simulink model "phdMain"  (R2023b)
settings: Solver=ode4  StartTime=0.0  StopTime=t.Data(end)  FixedStep=1e-3  RelTol=1e-3
values from neighbouring files (symbols this model uses):
  Am = T * Ac * inv(T)    [ref_model_mrac.m]
  Bm = T * Bc    [ref_model_mrac.m]
  Cm = eye(3)    [ref_model_mrac.m]
  Dm = zeros(3,1)    [ref_model_mrac.m]
undefined symbols (not defined in the file or in its folder): A_bar, AEFF, B_E, C_bar, C_T, Cd_neg, Cd_pos, DiscIntNeverNeededParam, Gamma, H, k, K, L_gain, L_STROKE, M, m3PsToLpm, P_return_Pa, P_supply_Pa, PA_Pa, PaToBar, PB_Pa, RHO, Ts, V01, V02, V_DEAD, v_mPs, W, xc_dot, xc_m
(part 2 of 3)

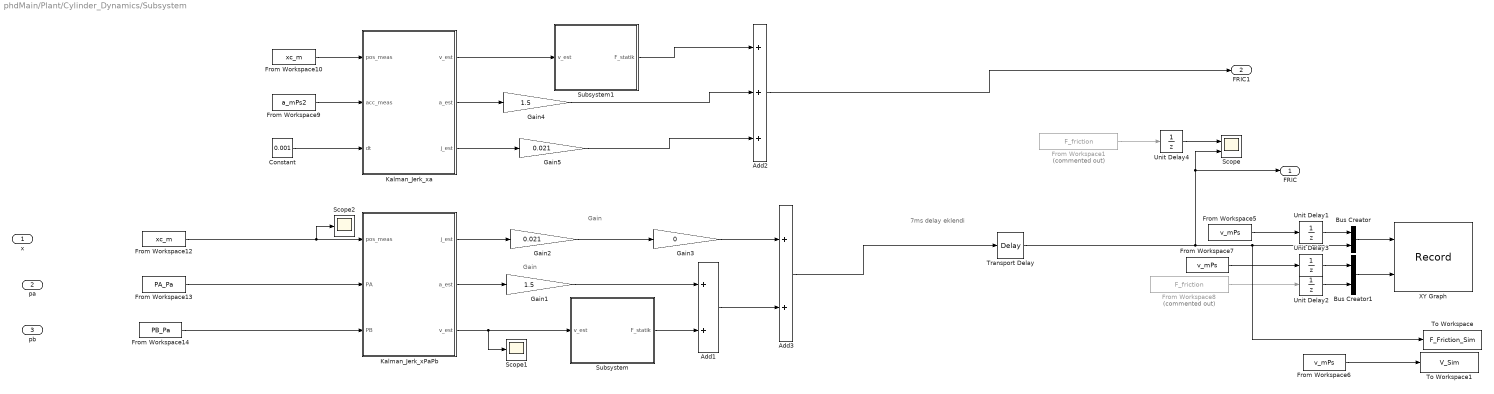
== system phdMain/Plant/Cylinder_Dynamics/Subsystem ==
  note: Gain
  note: 7ms delay eklendi
  note: Gain
  x : Inport
  pa : Inport  Port=2
  pb : Inport  Port=3
  Add1 : Sum
  Add2 : Sum  Inputs=+++
  Add3 : Sum
  Bus Creator : BusCreator  Inputs=2
  Bus Creator1 : BusCreator  Inputs=2
  Constant : Constant  Value=0.001
  From Workspace1 : FromWorkspace  Commented=on  VariableName=F_friction
  From Workspace10 : FromWorkspace  VariableName=xc_m
  From Workspace12 : FromWorkspace  VariableName=xc_m
  From Workspace13 : FromWorkspace  VariableName=PA_Pa
  From Workspace14 : FromWorkspace  VariableName=PB_Pa
  From Workspace5 : FromWorkspace  VariableName=v_mPs
  From Workspace6 : FromWorkspace  VariableName=v_mPs
  From Workspace7 : FromWorkspace  VariableName=v_mPs
  From Workspace8 : FromWorkspace  Commented=on  VariableName=F_friction
  From Workspace9 : FromWorkspace  VariableName=a_mPs2
  Gain1 : Gain  Gain=1.5
  Gain2 : Gain  Gain=0.021
  Gain3 : Gain  Gain=0
  Gain4 : Gain  Gain=1.5
  Gain5 : Gain  Gain=0.021
  Kalman_Jerk_xPaPb : MATLAB Function  TreatAsAtomicUnit=on
  Kalman_Jerk_xa : MATLAB Function  TreatAsAtomicUnit=on
  Scope : Scope  NumInputPorts=2
  Scope1 : Scope
  Scope2 : Scope
  Subsystem : Subsystem
  Subsystem1 : Subsystem
  To Workspace : ToWorkspace  VariableName=F_Friction_Sim  SaveFormat=Timeseries  SampleTime=-1
  To Workspace1 : ToWorkspace  VariableName=V_Sim  SaveFormat=Timeseries  SampleTime=-1
  Transport Delay : TransportDelay  DelayTime=7e-3
  Unit Delay{1..4} (4 alike) : UnitDelay  SampleTime=-1  HasFrameUpgradeWarning=on
  XY Graph : Record  FileSettingsInternal="{\"entries\":[{\"content\":{\"excelSettings\":{\"content\":{},\"type\":\"Streamout.ExcelSettings\"}},\"type\":\"Streamout.FileSettingStorage\",\"uuid\":\"\"}],\"packageUris\":[\"http:\\/\\/schema.mathworks.com\\/mf0\\/streamout_blocks\\/R2020a\"],\"version\":\"1.0\"}"  Layout=[1 1]  SignalsInternal="{\"entries\":[{\"content\":{\"signals\":[{\"content\":{\"blockPath\":[],\"dimensions\":[1],\"domain\":\"\",\"lineColor\":\"#0072bd\",\"port\":1,\"signalID\":19,\"signalName\":\"Bus Creator\"},\"type\":\"RecordBlkView.Signal\",\"uuid\":\"\"},{\"content\":{\"blockPath\":[],\"dimensions\":[1],\"domain\":\"\",\"lineColor\":\"#d95319\",\"port\":2,\"signalID\":22,\"signalName\":\"Bus Creator1\"},\"type\":\"RecordBlkView.Signal\",\"uuid\":\"\"}]},\"type\":\"RecordBlkView.InputSignals\",\"uuid\":\"\"}],\"packageUris\":[\"http:\\/\\/schema.mathworks.com\\/mf0\\/streamout_blocks\\/R2020a\"],\"version\":\"1.0\"}"  VisualizationBindings="{\"xyplotplugin\":{\"info\":[{\"series\":[],\"subplotID\":1}]}}"  CompatibilityTag=XY
  FRIC : Outport
  FRIC1 : Outport  Port=2
  wires:
  Unit Delay2/1 -> Bus Creator1/2
  From Workspace9/1 -> Kalman_Jerk_xa/2(acc_meas)
  Constant/1 -> Kalman_Jerk_xa/3(dt)
  From Workspace12/1 -> Scope2/1, Kalman_Jerk_xPaPb/1(pos_meas)
  From Workspace7/1 -> Unit Delay3/1
  Unit Delay3/1 -> Bus Creator1/1
  From Workspace13/1 -> Kalman_Jerk_xPaPb/2(PA)
  Add3/1 -> Transport Delay/1
  Bus Creator1/1 -> XY Graph/2
  From Workspace10/1 -> Kalman_Jerk_xa/1(pos_meas)
  From Workspace5/1 -> Unit Delay1/1
  Bus Creator/1 -> XY Graph/1
  From Workspace14/1 -> Kalman_Jerk_xPaPb/3(PB)
  Kalman_Jerk_xPaPb/1(j_est) -> Gain2/1
  From Workspace8/1 -> Unit Delay2/1
  Kalman_Jerk_xPaPb/2(a_est) -> Gain1/1
  From Workspace6/1 -> To Workspace1/1
  Unit Delay1/1 -> Bus Creator/1
  Kalman_Jerk_xPaPb/3(v_est) -> Scope1/1, Subsystem/1(v_est)
  From Workspace1/1 -> Unit Delay4/1
  Unit Delay4/1 -> Scope/1
  Transport Delay/1 -> Scope/2, FRIC/1, Bus Creator/2, To Workspace/1
  Subsystem/1(F_statik) -> Add1/2
  Gain1/1 -> Add1/1
  Gain2/1 -> Gain3/1
  Add1/1 -> Add3/2
  Gain3/1 -> Add3/1
  Kalman_Jerk_xa/2(a_est) -> Gain4/1
  Kalman_Jerk_xa/1(v_est) -> Subsystem1/1(v_est)
  Subsystem1/1(F_statik) -> Add2/1
  Gain4/1 -> Add2/2
  Add2/1 -> FRIC1/1
  Kalman_Jerk_xa/3(j_est) -> Gain5/1
  Gain5/1 -> Add2/3

== system phdMain/Plant/Cylinder_Dynamics/Subsystem1 ==
  Constant2 : Constant  Value=-0.09580
  Constant5 : Constant  Value=0.09580
  Constant6 : Constant  Value=1e6
  Constant7 : Constant  Value=2e-3
  MATLAB Function1 : MATLAB Function  TreatAsAtomicUnit=on
  F_end : Outport
  wires:
  Constant7/1 -> MATLAB Function1/6(v_lock)
  [xc_sim] -> MATLAB Function1/1(x)
  [xc_dot_sim] -> MATLAB Function1/2(x_dot)
  Constant6/1 -> MATLAB Function1/5(k_end)
  Constant2/1 -> MATLAB Function1/3(xmin)
  Constant5/1 -> MATLAB Function1/4(xmax)
  MATLAB Function1/1(F_end) -> F_end/1

== system phdMain/Subsystem2/Subsystem3/Subsystem ==
  y : Inport
  phi2_hat : Inport  Port=2
  d1_hat : Inport  Port=3
  l1 : Inport  Port=4
  eta : Inport  Port=5
  phi1_hat : Inport  Port=6
  Add : Sum  Inputs=+-
  Add1 : Sum
  Add2 : Sum
  Product : Product
  Product1 : Product
  phi1_hat_dot : Outport
  wires:
  eta/1 -> Product/2
  l1/1 -> Product/1
  phi1_hat/1 -> Add/2
  y/1 -> Add/1
  Product/1 -> Product1/1
  Add/1 -> Product1/2
  Product1/1 -> Add1/2
  d1_hat/1 -> Add1/1
  Add1/1 -> Add2/2
  phi2_hat/1 -> Add2/1
  Add2/1 -> phi1_hat_dot/1

== system phdMain/Subsystem2/Subsystem3/Subsystem1 ==
  phi1_hat : Inport
  d2_hat : Inport  Port=2
  l2 : Inport  Port=3
  eta : Inport  Port=4
  y : Inport  Port=5
  x3 : Inport  Port=6
  x4 : Inport  Port=7
  phi2_hat : Inport  Port=8
  Add : Sum  Inputs=+-
  Add1 : Sum
  Add2 : Sum
  Add3 : Sum  Inputs=+++
  Constant : Constant  Value=AEFF
  Constant1 : Constant  Value=M
  Divide : Product  Inputs=*/  RndMeth=Zero  SaturateOnIntegerOverflow=on
  Gain : Gain  Gain=1/M
  Lugre_Model : Subsystem
  Product{,1,3..4} (4 alike) : Product
  Unary Minus1 : UnaryMinus
  phi2_hat_dot : Outport
  wires:
  Add2/1 -> phi2_hat_dot/1
  Add1/1 -> Add2/2
  d2_hat/1 -> Add1/1
  Product1/1 -> Add1/2
  Add/1 -> Product1/2
  Product/1 -> Product1/1
  y/1 -> Add/1
  phi1_hat/1 -> Add/2
  l2/1 -> Product/1
  eta/1 -> Product/2
  Divide/1 -> Product3/1, Unary Minus1/1  "a23"
  x3/1 -> Product3/2
  Unary Minus1/1 -> Product4/1  "a24"
  x4/1 -> Product4/2
  Product3/1 -> Add3/2
  Product4/1 -> Add3/3
  Add3/1 -> Add2/1
  phi2_hat/1 -> Lugre_Model/1(xc_dot)
  Gain/1 -> Add3/1
  Lugre_Model/1(F_friction) -> Gain/1  "F_friction"
  Constant/1 -> Divide/1
  Constant1/1 -> Divide/2

== system phdMain/Subsystem2/Subsystem3/Subsystem3 ==
  phi2_hat : Inport
  gamma1 : Inport  Port=2
  phi1_hat : Inport  Port=3
  sigma1_hat : Inport  Port=4
  Add : Sum
  Add1 : Sum
  Product : Product
  Product1 : Product
  Unary Minus : UnaryMinus
  sigma1_hat_dot : Outport
  wires:
  sigma1_hat/1 -> Add/1
  Product/1 -> Add/2
  Add/1 -> Add1/2
  phi2_hat/1 -> Add1/1
  gamma1/1 -> Unary Minus/1, Product/2
  phi1_hat/1 -> Product/1
  Add1/1 -> Product1/1
  Unary Minus/1 -> Product1/2
  Product1/1 -> sigma1_hat_dot/1

== system phdMain/Subsystem2/Subsystem3/Subsystem4 ==
  phi2_hat : Inport
  gamma2 : Inport  Port=2
  x3 : Inport  Port=3
  x4 : Inport  Port=4
  sigma2_hat : Inport  Port=5
  Add : Sum
  Add2 : Sum
  Add3 : Sum  Inputs=+++
  Constant : Constant  Value=AEFF
  Constant1 : Constant  Value=M
  Divide : Product  Inputs=*/  RndMeth=Zero  SaturateOnIntegerOverflow=on
  Gain : Gain  Gain=1/M
  Lugre_Model : Subsystem
  Product{,1,3..4} (4 alike) : Product
  Unary Minus : UnaryMinus
  Unary Minus1 : UnaryMinus
  sigma2_hat_dot : Outport
  wires:
  Product1/1 -> sigma2_hat_dot/1
  gamma2/1 -> Unary Minus/1, Product/2
  Product/1 -> Add/2
  sigma2_hat/1 -> Add/1
  Product3/1 -> Add3/2
  Product4/1 -> Add3/3
  x4/1 -> Product4/2
  phi2_hat/1 -> Product/1, Lugre_Model/1(xc_dot)
  Unary Minus1/1 -> Product4/1  "a24"
  x3/1 -> Product3/2
  Add3/1 -> Add2/1
  Gain/1 -> Add3/1
  Add/1 -> Add2/2
  Add2/1 -> Product1/1
  Unary Minus/1 -> Product1/2
  Lugre_Model/1(F_friction) -> Gain/1  "F_friction"
  Constant/1 -> Divide/1
  Divide/1 -> Product3/1, Unary Minus1/1  "a23"
  Constant1/1 -> Divide/2

== system phdMain/Subsystem2/Subsystem3/Subsystem6 ==
  sigma1_hat : Inport
  gamma1 : Inport  Port=2
  phi1_hat : Inport  Port=3
  Add : Sum
  Product : Product
  d1_hat : Outport
  wires:
  sigma1_hat/1 -> Add/1
  gamma1/1 -> Product/1
  phi1_hat/1 -> Product/2
  Product/1 -> Add/2
  Add/1 -> d1_hat/1

== system phdMain/Subsystem2/Subsystem3/Subsystem7 ==
  sigma2_hat : Inport
  gamma2 : Inport  Port=2
  phi2_hat : Inport  Port=3
  Add : Sum
  Product : Product
  d2_hat : Outport
  wires:
  gamma2/1 -> Product/1
  sigma2_hat/1 -> Add/1
  Product/1 -> Add/2
  Add/1 -> d2_hat/1
  phi2_hat/1 -> Product/2

== system phdMain/old/Flow_Calc_NoLeak/Subsystem1 ==
  Constant : Constant  Value=Cd_pos
  Constant1 : Constant  Value=W
  Constant2 : Constant  Value=RHO
  Constant3 : Constant  Value=2
  Math Reciprocal : Math  Operator=reciprocal  SignedPower=on
  Product : Product  Inputs=3
  Product1 : Product
  Sqrt : Sqrt
  Kq : Outport
  wires:
  Product/1 -> Kq/1
  Sqrt/1 -> Product/3
  Product1/1 -> Sqrt/1
  Constant3/1 -> Product1/1
  Math Reciprocal/1 -> Product1/2
  Constant2/1 -> Math Reciprocal/1  "rho"
  Constant1/1 -> Product/2  "w"
  Constant/1 -> Product/1  "Cd"

== system phdMain/old/Flow_Calc_NoLeak/Subsystem2 ==
  Constant : Constant  Value=Cd_neg
  Constant1 : Constant  Value=W
  Constant2 : Constant  Value=RHO
  Constant3 : Constant  Value=2
  Math Reciprocal : Math  Operator=reciprocal  SignedPower=on
  Product : Product  Inputs=3
  Product1 : Product
  Sqrt : Sqrt
  Kq : Outport
  wires:
  Constant/1 -> Product/1  "Cd"
  Constant1/1 -> Product/2  "w"
  Constant2/1 -> Math Reciprocal/1  "rho"
  Math Reciprocal/1 -> Product1/2
  Constant3/1 -> Product1/1
  Product1/1 -> Sqrt/1
  Sqrt/1 -> Product/3
  Product/1 -> Kq/1

== system phdMain/old/ServoValve_Dynamics/Convert_SpoolPosition ==
  u_perc : Inport  OutDataTypeStr=double
  Constant : Constant  Value=50e-3
  Constant1 : Constant  Value=0.01
  Constant2 : Constant  Value=0.001016
  Constant3 : Constant  Value=50e-3
  Math Reciprocal : Math  Operator=reciprocal  SignedPower=on
  Product : Product  Inputs=3
  Product1 : Product
  Product2 : Product
  xv : Outport  OutDataTypeStr=double
  wires:
  u_perc/1 -> Product/3
  Constant1/1 -> Product/2
  Constant3/1 -> Product/1
  Constant2/1 -> Product1/1
  Math Reciprocal/1 -> Product1/2
  Constant/1 -> Math Reciprocal/1
  Product1/1 -> Product2/2  "Ki"
  Product/1 -> Product2/1  "i"
  Product2/1 -> xv/1  "xv"

== system phdMain/old/ServoValve_Dynamics/Subsystem ==
  Valve Dynamics1 : TransferFcn  Numerator=[7.738e05]  Denominator=[1 1244 7.738e05]
  Valve Dynamics2 : TransferFcn  Numerator=[(120*2*pi)^2]  Denominator=[1 2*0.95*(120*2*pi) (120*2*pi)^2]

== system phdMain/Nguyen Observer/Nguyen_Observer/phi_calc/Delta_1 ==
  x1 : Inport
  Add2 : Sum
  Constant5 : Constant  Value=B_E
  Constant6 : Constant  Value=AEFF
  Constant7 : Constant  Value=V01
  Gain : Gain  Gain=1e-2
  Math Reciprocal : Math  Operator=reciprocal  SignedPower=on
  Product5 : Product
  Product6 : Product
  Delta_1 : Outport
  wires:
  Product5/1 -> Add2/2
  Constant5/1 -> Gain/1
  Math Reciprocal/1 -> Product6/2
  x1/1 -> Product5/2
  Product6/1 -> Delta_1/1
  Add2/1 -> Math Reciprocal/1
  Constant6/1 -> Product5/1
  Constant7/1 -> Add2/1
  Gain/1 -> Product6/1

== system phdMain/Nguyen Observer/Nguyen_Observer/phi_calc/Delta_2 ==
  x1 : Inport
  Add2 : Sum  Inputs=+-
  Constant5 : Constant  Value=B_E
  Constant6 : Constant  Value=AEFF
  Constant7 : Constant  Value=V02
  Gain2 : Gain  Gain=1e-2
  Math Reciprocal : Math  Operator=reciprocal  SignedPower=on
  Product5 : Product
  Product6 : Product
  Delta_2 : Outport
  wires:
  Add2/1 -> Math Reciprocal/1
  Product6/1 -> Delta_2/1
  x1/1 -> Product5/2
  Math Reciprocal/1 -> Product6/2
  Constant5/1 -> Gain2/1
  Product5/1 -> Add2/2
  Constant6/1 -> Product5/1
  Constant7/1 -> Add2/1
  Gain2/1 -> Product6/1

== system phdMain/Plant/Cylinder_Dynamics/Lugre_Model/Subsystem1 ==
  term : Inport
  z_prev : Inport  Port=2
  v : Inport  Port=3
  Add : Sum
  Add1 : Sum
  Constant : Constant
  Gain : Gain  Gain=1e-3
  Gain1 : Gain  Gain=1e-3
  Math Reciprocal2 : Math  Operator=reciprocal  SignedPower=on
  Product : Product
  z : Outport
  wires:
  term/1 -> Gain1/1
  z_prev/1 -> Add/1
  v/1 -> Gain/1
  Gain/1 -> Add/2
  Add/1 -> Product/1
  Gain1/1 -> Add1/2
  Constant/1 -> Add1/1
  Add1/1 -> Math Reciprocal2/1
  Math Reciprocal2/1 -> Product/2
  Product/1 -> z/1

== system phdMain/Plant/Cylinder_Dynamics/Subsystem/Subsystem ==
  v_est : Inport
  MATLAB Function : MATLAB Function  TreatAsAtomicUnit=on
  F_statik : Outport
  wires:
  v_est/1 -> MATLAB Function/1(v)
  MATLAB Function/1(F_statik) -> F_statik/1

== system phdMain/Plant/Cylinder_Dynamics/Subsystem/Subsystem1 ==
  v_est : Inport
  MATLAB Function : MATLAB Function  TreatAsAtomicUnit=on
  F_statik : Outport
  wires:
  MATLAB Function/1(F_statik) -> F_statik/1
  v_est/1 -> MATLAB Function/1(v)

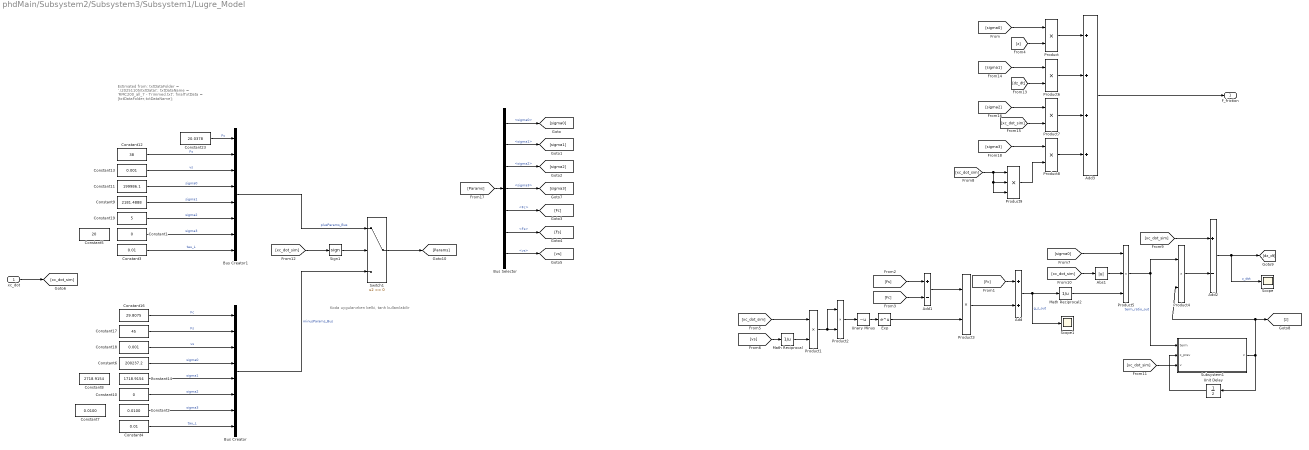
== system phdMain/Subsystem2/Subsystem3/Subsystem1/Lugre_Model ==
  note: Koda uygulanırken belki, tanh kullanılabilir
  note: Estimated from:
      |
      | txtDataFolder = '.\20251105\txtData\';
      | txtDataName = 'RMC200_all_7 - Trimmed.txt';
      | finalTxtData = [txtDataFolder,txtDataName];
  xc_dot : Inport  OutDataTypeStr=double
  Abs1 : Abs  SaturateOnIntegerOverflow=off
  Add : Sum
  Add1 : Sum  Inputs=+-
  Add2 : Sum  Inputs=+-
  Add3 : Sum  Inputs=++++
  Bus Selector : BusSelector  OutputSignals=sigma0,sigma1,sigma2,sigma3,Fc,Fs,vs
  Bus Creator : BusCreator  Inputs=8
  Bus Creator1 : BusCreator  Inputs=8
  Constant1 : Constant  Value=0  OutDataTypeStr=double
  Constant10 : Constant  Value=0  OutDataTypeStr=double
  Constant11 : Constant  Value=199986.1  OutDataTypeStr=double
  Constant12 : Constant  Value=38  OutDataTypeStr=double
  Constant13 : Constant  Value=0.001  OutDataTypeStr=double
  Constant14 : Constant  Value=1718.9154  OutDataTypeStr=double
  Constant16 : Constant  Value=29.8075  OutDataTypeStr=double
  Constant17 : Constant  Value=45  OutDataTypeStr=double
  Constant18 : Constant  Value=0.001  OutDataTypeStr=double
  Constant19 : Constant  Value=5  OutDataTypeStr=double
  Constant2 : Constant  Value=0.0100  OutDataTypeStr=double
  Constant23 : Constant  Value=20.0378  OutDataTypeStr=double
  Constant3 : Constant  Value=0.01  OutDataTypeStr=double
  Constant4 : Constant  Value=0.01  OutDataTypeStr=double
  Constant5 : Constant  Value=20  OutDataTypeStr=double
  Constant6 : Constant  Value=200237.2  OutDataTypeStr=double
  Constant7 : Constant  Value=0.0100  OutDataTypeStr=double
  Constant8 : Constant  Value=2718.9154  OutDataTypeStr=double
  Constant9 : Constant  Value=2181.4888  OutDataTypeStr=double
  Exp : Math  SignedPower=on
  Math Reciprocal : Math  Operator=reciprocal  SignedPower=on
  Math Reciprocal2 : Math  Operator=reciprocal  SignedPower=on
  Product{,1..4,6..8} (8 alike) : Product
  Product5 : Product  Inputs=3
  Product9 : Product  Inputs=3
  Scope : Scope
  Scope1 : Scope
  Sign1 : Signum
  Subsystem1 : Subsystem
  Switch1 : Switch  SaturateOnIntegerOverflow=off  InputSameDT=off
  Unary Minus : UnaryMinus
  Unit Delay : UnitDelay  SampleTime=-1  HasFrameUpgradeWarning=on
  F_friction : Outport
  wires:
  Constant18/1 -> Bus Creator/3  "vs"
  Constant13/1 -> Bus Creator1/3  "vs"
  Constant12/1 -> Bus Creator1/2  "Fs"
  Constant17/1 -> Bus Creator/2  "Fs"
  Constant14/1 -> Bus Creator/5  "sigma1"
  Constant6/1 -> Bus Creator/4  "sigma0"
  Constant10/1 -> Bus Creator/6  "sigma2"
  Constant16/1 -> Bus Creator/1  "Fc"
  Constant9/1 -> Bus Creator1/5  "sigma1"
  Constant11/1 -> Bus Creator1/4  "sigma0"
  Constant19/1 -> Bus Creator1/6  "sigma2"
  Product7/1 -> Add3/3
  Product6/1 -> Add3/2
  [sigma2] -> Product7/1
  [xc_dot_sim] -> Product7/2
  [dz_dt] -> Product6/2
  [sigma1] -> Product6/1
  Product/1 -> Add3/1
  [z] -> Product/2
  [sigma0] -> Product5/1
  Abs1/1 -> Product5/2
  Add/1 -> Math Reciprocal2/1, Scope1/1  "g_s_out"
  [xc_dot_sim] -> Abs1/1
  Add1/1 -> Product3/1
  Unary Minus/1 -> Exp/1
  Product2/1 -> Unary Minus/1
  Product1/1 -> Product2/2, Product2/1
  [xc_dot_sim] -> Product1/1
  Math Reciprocal/1 -> Product1/2
  [vs] -> Math Reciprocal/1
  [Fc] -> Add1/2
  [Fs] -> Add1/1
  [Fc] -> Add/1
  [sigma0] -> Product/1
  Product3/1 -> Add/2
  [xc_dot_sim] -> Sign1/1
  Bus Creator1/1 -> Switch1/1  "plusParams_Bus"
  Bus Creator/1 -> Switch1/3  "minusParams_Bus"
  Switch1/1 -> [Params]
  [Params] -> Bus Selector/1
  Bus Selector/1 -> [sigma0]  "<sigma0>"
  Bus Selector/2 -> [sigma1]  "<sigma1>"
  Bus Selector/3 -> [sigma2]  "<sigma2>"
  Bus Selector/5 -> [Fc]  "<Fc>"
  Bus Selector/6 -> [Fs]  "<Fs>"
  Bus Selector/7 -> [vs]  "<vs>"
  Math Reciprocal2/1 -> Product5/3
  Exp/1 -> Product3/2
  Add2/1 -> Scope/1, [dz_dt]  "z_dot"
  Sign1/1 -> Switch1/2
  [xc_dot_sim] -> Add2/1
  Subsystem1/1(z) -> Product4/2, [z], Unit Delay/1
  [xc_dot_sim] -> Subsystem1/3(v)
  Unit Delay/1 -> Subsystem1/2(z_prev)
  Product5/1 -> Subsystem1/1(term), Product4/1  "term_ratio_out"
  Product4/1 -> Add2/2
  Add3/1 -> F_friction/1
  Constant1/1 -> Bus Creator1/7  "sigma3"
  Constant2/1 -> Bus Creator/7  "sigma3"
  Constant3/1 -> Bus Creator1/8  "tau_L"
  Constant4/1 -> Bus Creator/8  "tau_L"
  [sigma3] -> Product8/1
  Product8/1 -> Add3/4
  [xc_dot_sim] -> Product9/2, Product9/3, Product9/1
  Product9/1 -> Product8/2
  Bus Selector/4 -> [sigma3]  "<sigma3>"
  xc_dot/1 -> [xc_dot_sim]
  Constant23/1 -> Bus Creator1/1  "Fc"

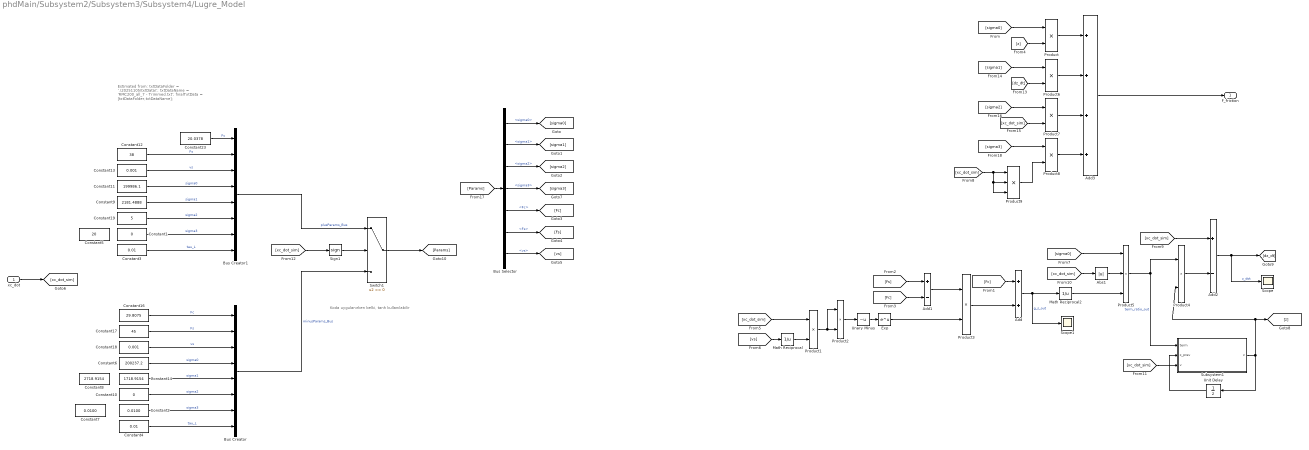
== system phdMain/Subsystem2/Subsystem3/Subsystem4/Lugre_Model ==
  note: Koda uygulanırken belki, tanh kullanılabilir
  note: Estimated from:
      |
      | txtDataFolder = '.\20251105\txtData\';
      | txtDataName = 'RMC200_all_7 - Trimmed.txt';
      | finalTxtData = [txtDataFolder,txtDataName];
  xc_dot : Inport  OutDataTypeStr=double
  Abs1 : Abs  SaturateOnIntegerOverflow=off
  Add : Sum
  Add1 : Sum  Inputs=+-
  Add2 : Sum  Inputs=+-
  Add3 : Sum  Inputs=++++
  Bus Selector : BusSelector  OutputSignals=sigma0,sigma1,sigma2,sigma3,Fc,Fs,vs
  Bus Creator : BusCreator  Inputs=8
  Bus Creator1 : BusCreator  Inputs=8
  Constant1 : Constant  Value=0  OutDataTypeStr=double
  Constant10 : Constant  Value=0  OutDataTypeStr=double
  Constant11 : Constant  Value=199986.1  OutDataTypeStr=double
  Constant12 : Constant  Value=38  OutDataTypeStr=double
  Constant13 : Constant  Value=0.001  OutDataTypeStr=double
  Constant14 : Constant  Value=1718.9154  OutDataTypeStr=double
  Constant16 : Constant  Value=29.8075  OutDataTypeStr=double
  Constant17 : Constant  Value=45  OutDataTypeStr=double
  Constant18 : Constant  Value=0.001  OutDataTypeStr=double
  Constant19 : Constant  Value=5  OutDataTypeStr=double
  Constant2 : Constant  Value=0.0100  OutDataTypeStr=double
  Constant23 : Constant  Value=20.0378  OutDataTypeStr=double
  Constant3 : Constant  Value=0.01  OutDataTypeStr=double
  Constant4 : Constant  Value=0.01  OutDataTypeStr=double
  Constant5 : Constant  Value=20  OutDataTypeStr=double
  Constant6 : Constant  Value=200237.2  OutDataTypeStr=double
  Constant7 : Constant  Value=0.0100  OutDataTypeStr=double
  Constant8 : Constant  Value=2718.9154  OutDataTypeStr=double
  Constant9 : Constant  Value=2181.4888  OutDataTypeStr=double
  Exp : Math  SignedPower=on
  Math Reciprocal : Math  Operator=reciprocal  SignedPower=on
  Math Reciprocal2 : Math  Operator=reciprocal  SignedPower=on
  Product{,1..4,6..8} (8 alike) : Product
  Product5 : Product  Inputs=3
  Product9 : Product  Inputs=3
  Scope : Scope
  Scope1 : Scope
  Sign1 : Signum
  Subsystem1 : Subsystem
  Switch1 : Switch  SaturateOnIntegerOverflow=off  InputSameDT=off
  Unary Minus : UnaryMinus
  Unit Delay : UnitDelay  SampleTime=-1  HasFrameUpgradeWarning=on
  F_friction : Outport
  wires:
  Constant18/1 -> Bus Creator/3  "vs"
  Constant13/1 -> Bus Creator1/3  "vs"
  Constant12/1 -> Bus Creator1/2  "Fs"
  Constant17/1 -> Bus Creator/2  "Fs"
  Constant14/1 -> Bus Creator/5  "sigma1"
  Constant6/1 -> Bus Creator/4  "sigma0"
  Constant10/1 -> Bus Creator/6  "sigma2"
  Constant16/1 -> Bus Creator/1  "Fc"
  Constant9/1 -> Bus Creator1/5  "sigma1"
  Constant11/1 -> Bus Creator1/4  "sigma0"
  Constant19/1 -> Bus Creator1/6  "sigma2"
  Product7/1 -> Add3/3
  Product6/1 -> Add3/2
  [sigma2] -> Product7/1
  [xc_dot_sim] -> Product7/2
  [dz_dt] -> Product6/2
  [sigma1] -> Product6/1
  Product/1 -> Add3/1
  [z] -> Product/2
  [sigma0] -> Product5/1
  Abs1/1 -> Product5/2
  Add/1 -> Math Reciprocal2/1, Scope1/1  "g_s_out"
  [xc_dot_sim] -> Abs1/1
  Add1/1 -> Product3/1
  Unary Minus/1 -> Exp/1
  Product2/1 -> Unary Minus/1
  Product1/1 -> Product2/2, Product2/1
  [xc_dot_sim] -> Product1/1
  Math Reciprocal/1 -> Product1/2
  [vs] -> Math Reciprocal/1
  [Fc] -> Add1/2
  [Fs] -> Add1/1
  [Fc] -> Add/1
  [sigma0] -> Product/1
  Product3/1 -> Add/2
  [xc_dot_sim] -> Sign1/1
  Bus Creator1/1 -> Switch1/1  "plusParams_Bus"
  Bus Creator/1 -> Switch1/3  "minusParams_Bus"
  Switch1/1 -> [Params]
  [Params] -> Bus Selector/1
  Bus Selector/1 -> [sigma0]  "<sigma0>"
  Bus Selector/2 -> [sigma1]  "<sigma1>"
  Bus Selector/3 -> [sigma2]  "<sigma2>"
  Bus Selector/5 -> [Fc]  "<Fc>"
  Bus Selector/6 -> [Fs]  "<Fs>"
  Bus Selector/7 -> [vs]  "<vs>"
  Math Reciprocal2/1 -> Product5/3
  Exp/1 -> Product3/2
  Add2/1 -> Scope/1, [dz_dt]  "z_dot"
  Sign1/1 -> Switch1/2
  [xc_dot_sim] -> Add2/1
  Subsystem1/1(z) -> Product4/2, [z], Unit Delay/1
  [xc_dot_sim] -> Subsystem1/3(v)
  Unit Delay/1 -> Subsystem1/2(z_prev)
  Product5/1 -> Subsystem1/1(term), Product4/1  "term_ratio_out"
  Product4/1 -> Add2/2
  Add3/1 -> F_friction/1
  Constant1/1 -> Bus Creator1/7  "sigma3"
  Constant2/1 -> Bus Creator/7  "sigma3"
  Constant3/1 -> Bus Creator1/8  "tau_L"
  Constant4/1 -> Bus Creator/8  "tau_L"
  [sigma3] -> Product8/1
  Product8/1 -> Add3/4
  [xc_dot_sim] -> Product9/2, Product9/3, Product9/1
  Product9/1 -> Product8/2
  Bus Selector/4 -> [sigma3]  "<sigma3>"
  xc_dot/1 -> [xc_dot_sim]
  Constant23/1 -> Bus Creator1/1  "Fc"

== system phdMain/Subsystem2/Subsystem3/Subsystem1/Lugre_Model/Subsystem1 ==
  term : Inport
  z_prev : Inport  Port=2
  v : Inport  Port=3
  Add : Sum
  Add1 : Sum
  Constant : Constant
  Gain : Gain  Gain=1e-3
  Gain1 : Gain  Gain=1e-3
  Math Reciprocal2 : Math  Operator=reciprocal  SignedPower=on
  Product : Product
  z : Outport
  wires:
  term/1 -> Gain1/1
  z_prev/1 -> Add/1
  v/1 -> Gain/1
  Gain/1 -> Add/2
  Add/1 -> Product/1
  Gain1/1 -> Add1/2
  Constant/1 -> Add1/1
  Add1/1 -> Math Reciprocal2/1
  Math Reciprocal2/1 -> Product/2
  Product/1 -> z/1

== system phdMain/Subsystem2/Subsystem3/Subsystem4/Lugre_Model/Subsystem1 ==
  term : Inport
  z_prev : Inport  Port=2
  v : Inport  Port=3
  Add : Sum
  Add1 : Sum
  Constant : Constant
  Gain : Gain  Gain=1e-3
  Gain1 : Gain  Gain=1e-3
  Math Reciprocal2 : Math  Operator=reciprocal  SignedPower=on
  Product : Product
  z : Outport
  wires:
  term/1 -> Gain1/1
  z_prev/1 -> Add/1
  v/1 -> Gain/1
  Gain/1 -> Add/2
  Add/1 -> Product/1
  Gain1/1 -> Add1/2
  Constant/1 -> Add1/1
  Add1/1 -> Math Reciprocal2/1
  Math Reciprocal2/1 -> Product/2
  Product/1 -> z/1

== matlab function phdMain/Plant/Cylinder_Dynamics/Subsystem/Kalman_Jerk_xa ==
  settings: updateMethod=DISCRETE
  data: pos_meas input; v_est output; acc_meas input; dt input; a_est output; j_est output
function [v_est, a_est, j_est] = fcn(pos_meas, acc_meas, dt)
    % KALMAN FİLTRESİ (Jerk Augmented)
    % Durumlar: x = [Pozisyon; Hız; İvme; Jerk]
    
    % Değişkenleri hafızada tutmak için 'persistent' tanımlıyoruz
    persistent x P A H Q R I initialized
    
    % --- BAŞLANGIÇ AYARLARI (Sadece ilk adımda çalışır) ---
    if isempty(initialized)
        % Başlangıç Durumu (İlk ölçüme göre)
        x = [pos_meas; 0; acc_meas; 0]; 
        
        % Başlangıç Belirsizliği
        P = eye(4); 
        
        % Matris Tanımları (Sabitler)
        % 1. Geçiş Matrisi (Fizik: x = x0 + v*dt + 0.5*a*dt^2 + ...)
        A = [1, dt, 0.5*dt^2, (1/6)*dt^3;
             0,  1,       dt,   0.5*dt^2;
             0,  0,        1,         dt;
             0,  0,        0,          1];
         
        % 2. Ölçüm Matrisi (Sadece Pos ve Acc ölçüyoruz)
        H = [1, 0, 0, 0;
             0, 0, 1, 0];
         
        % 3. Gürültü Kovaryansları (TUNING BURADAN)
        sigma_jerk = 2000; % Sistemin vahşiliği (Spike yakalama yeteneği)
        
        % Q (Süreç Gürültüsü)
        Q = diag([dt^6/36, dt^4/4, dt^2, 1]) * sigma_jerk^2;
        
        % R (Ölçüm Gürültüsü) - Sensör güveni
        R_pos = (1e-6)^2;
        R_acc = (0.5)^2;
        R = diag([R_pos, R_acc]);
        
        I = eye(4);
        initialized = 1;
    end
    
    % --- KALMAN DÖNGÜSÜ (Her adımda çalışır) ---
    
    % 1. PREDICT (Öngörü)
    x_pred = A * x;
    P_pred = A * P * A' + Q;
    
    % 2. UPDATE (Düzeltme)
    z = [pos_meas; acc_meas]; % Ölçüm vektörü
    
    y = z - H * x_pred;       % Innovation (Hata)
    S = H * P_pred * H' + R;  % Innovation Covaryans
    K = P_pred * H' / S;      % Kalman Kazancı
    
    x = x_pred + K * y;       % Durum Güncelleme
    P = (I - K * H) * P_pred; % Kovaryans Güncelleme
    
    % 3. ÇIKTI
    v_est = x(2);
    a_est = x(3);
    j_est = x(4);
end

== matlab function phdMain/Plant/Cylinder_Dynamics/Subsystem/Kalman_Jerk_xPaPb ==
  settings: updateMethod=DISCRETE
  data: j_est output; a_est output; pos_meas input; v_est output; PA input; PB input
function [j_est, a_est, v_est] = fcn(pos_meas, PA, PB)
    % PRESSURE-AIDED JERK ESTIMATOR
    % Girdiler: Pozisyon ve Basınçlar
    % Çıktı: Tertemiz Jerk (j_est)
    
    persistent x P A H Q R I initialized m AA AB
    
    % --- SABİTLER ---
    dt = 0.001;   % Örnekleme Zamanı (Simulink step size ile aynı olmalı)
    
    if isempty(initialized)
        % 1. SİSTEM TANIMLAMALARI
        m  = 3.4;       % Tahmini Hareketli Kütle (kg)
        AA = 2.0106e-04;  % A Odası Alanı (m2)
        AB = 2.0106e-04;  % B Odası Alanı (m2)
        
        % 2. DURUM VEKTÖRÜ: x = [Konum; Hız; İvme; Jerk]
        % (Sürtünme değil, doğrudan kinematiği izliyoruz)
        F_net_start = (PA*AA - PB*AB);
        a_start = F_net_start / m;
        
        x = [pos_meas; 0; a_start; 0];
        P = eye(4);
        I = eye(4);
        
        % 3. GEÇİŞ MATRİSİ (Constant Jerk Model)
        % x(k+1) = x(k) + v*dt + 0.5*a*dt^2 + 1/6*j*dt^3 ...
        A = [1, dt, 0.5*dt^2, (1/6)*dt^3;
             0,  1,       dt,   0.5*dt^2;
             0,  0,        1,         dt;
             0,  0,        0,          1];
         
        % 4. ÖLÇÜM MATRİSİ
        % z1 = Konum (x1)
        % z2 = İvme  (x3) -> Basınçtan türetilmiş "Sanal İvme"
        H = [1, 0, 0, 0;
             0, 0, 1, 0];
         
        % 5. TUNING (AYARLAR)
        % Q: Jerk ne kadar hızlı değişebilir? (Sistemin vahşiliği)
        % Yüksek değer = Zıplamaları anında yakalar (Gecikmesiz).
        sigma_jerk = 100; 
        Q = diag([dt^6/36, dt^4/4, dt^2, 1]) * sigma_jerk^2;
        
        % R: Ölçümlere ne kadar güveniyoruz?
        R_pos = (1e-6)^2; % Konum çok hassas
        R_acc = (2.0)^2;  % Basınçtan gelen ivme "gürültülüdür" (Sürtünme yok sayıldığı için)
                          % Burayı gevşek bırakıyoruz ki Kalman, konum verisiyle
                          % basınç verisini harmanlayıp doğruyu bulsun.
        R = diag([R_pos, R_acc]);
        
        initialized = 1;
    end
    
    % --- 1. SANAL İVME ÖLÇÜMÜ OLUŞTURMA ---
    % Basınç kuvvetini kütleye bölerek "Ham İvme" elde ediyoruz.
    % Not: Bu ivme sürtünmeyi içermez, bu yüzden "gürültülü/hatalı" kabul edilir.
    % Kalman bunu düzeltecek.
    F_hyd = PA * AA - PB * AB;
    a_meas_virtual = F_hyd / m; 
    
    % Ölçüm Vektörü
    z = [pos_meas; a_meas_virtual];
    
    % --- 2. KALMAN PREDICT ---
    x_pred = A * x;
    P_pred = A * P * A' + Q;
    
    % --- 3. KALMAN UPDATE ---
    y = z - H * x_pred;       % Hata (Innovation)
    S = H * P_pred * H' + R;  % Kovaryans
    K = P_pred * H' / S;      % Kazanç (Gain)
    
    x = x_pred + K * y;       % Güncelleme
    P = (I - K * H) * P_pred;
    
    % --- 4. ÇIKTILAR ---
    v_est = x(2);
    a_est = x(3);
    j_est = x(4); % İŞTE ARADIĞIN JERK!
end

== matlab function phdMain/Plant/Cylinder_Dynamics/Subsystem/Subsystem1/MATLAB Function ==
  data: v input; F_statik output
function F_statik = fcn(v)
Fc = 18; 
Fs = 75; 
v_s = 0.016; 
C = 100; 

F_statik = Fc + (Fs - Fc)*exp(-(1*abs(v)./v_s)^2);
F_statik = F_statik * tanh(C*v);

== matlab function phdMain/Plant/Cylinder_Dynamics/MATLAB Function1 ==
  data: v input; FF output; a input; j input
function FF = fcn(v,a,j)
% --- Geçiş Yumuşaklığı Parametresi ---
% Bu değer büyüdükçe 0'daki eğim azalır (daha eğimli geçer)
eps_smooth = 0.00223;


% --- Pozitif Yön (v > 0) ---
kv_p = 39.658; Fc_p = 25; Fs_p = 82.9; tau_p = 0.0016;

% --- Negatif Yön (v < 0) ---
kv_n = 38.5; Fc_n = 5; Fs_n = 75.17; tau_n = 0.0016;

% Yumuşatılmış yön fonksiyonu (sign yerine tanh)
% Bu fonksiyon -1 ile 1 arasında yumuşak bir geçiş sağlar
smooth_sign = tanh(v ./ eps_smooth);

% Asimetrik katsayı vektörleri oluşturma
% Hızın yönüne göre katsayıları seçiyoruz
kv = (v >= 0)*kv_p + (v < 0)*kv_n;
Fc = (v >= 0)*Fc_p + (v < 0)*Fc_n;
Fs = (v >= 0)*Fs_p + (v < 0)*Fs_n;
tau = (v >= 0)*tau_p + (v < 0)*tau_n;

F_stribeck = (kv .* v) + (Fc .* smooth_sign) + (Fs .* smooth_sign .* exp(-abs(v./tau)));

K_acc = 1.121235; 
K_jerk = 0.056481; 
kappa_delay = 0; 

FF = F_stribeck + K_acc * a  +  K_jerk*j;

== matlab function phdMain/Plant/Cylinder_Dynamics/MATLAB Function3 ==
  data: v input; F_friction_nodelay output; FF input; j input; a input
function F_friction_nodelay = fcn(v, FF, j, a)

K_acc_p = 1.021235; 
K_acc_n = 0.0810121235; 

K_jerk_p = -0.05656481; 
K_jerk_n = 0.02056481; 

K_acc = (v>=0)*K_acc_p + (v<0)*K_acc_n; 
K_jerk = (v>=0)*K_jerk_p + (v<0)*K_jerk_n; 

F_friction_nodelay = FF + K_acc .* a  +  K_jerk.*j;

== matlab function phdMain/Plant/Cylinder_Dynamics/MATLAB Function4 ==
  data: v input; F_stribeck output
function F_stribeck = fcn(v)


% close all 

% --- Geçiş Yumuşaklığı Parametresi ---
% Bu değer büyüdükçe 0'daki eğim azalır (daha eğimli geçer)
eps_smooth = 0.0223;
% eps_smooth = 0.015;

%%%
kv_p = 12; Fc_p = 25; Fs_p  = 383; tau_p = 0.016;
kv_n = 35; Fc_n = 7.5; Fs_n = 183; tau_n = 0.02016;
%%%


% Yumuşatılmış yön fonksiyonu (sign yerine tanh)
% Bu fonksiyon -1 ile 1 arasında yumuşak bir geçiş sağlar
smooth_sign = tanh(v ./ eps_smooth);

% Asimetrik katsayı vektörleri oluşturma
% Hızın yönüne göre katsayıları seçiyoruz
kv = (v >= 0)*kv_p + (v < 0)*kv_n;
Fc = (v >= 0)*Fc_p + (v < 0)*Fc_n;
Fs = (v >= 0)*Fs_p + (v < 0)*Fs_n;
tau = (v >= 0)*tau_p + (v < 0)*tau_n;
F_stribeck = (kv .* v) + (Fc .* smooth_sign) + (Fs .* smooth_sign .* exp(-abs(v./tau)));

== matlab function phdMain/Nguyen Observer/Nguyen_Observer/phi_calc/MATLAB Function ==
  data: Q1 output; Q2 output; u input; Ps input; Pr input; P1 input; P2 input; QR output
function [Q1, Q2, QR] = fcn(u, Ps, Pr, P1, P2)
    % x0 parametresini girişten kaldırdık, içeride asimetrik tanımlayacağız.
    % Valve params 
    K           = 0.00000334; 
    k           = 1.82709080; 

    % --- ASİMETRİK SIZINTI AYARLARI ---
    % Hedef: P_null = 70 bar (Ps=210 bar iken)
    % Bu dengeyi sağlamak için Return tarafı açıklığı daha büyük olmalı.

    % --- GÜNCELLENMİŞ ASİMETRİK SIZINTI AYARLARI ---
    % Hedef: Ps=200 bar, Pr=4.5 bar iken yaklaşık 70-75 bar denge basıncı
    % $$x_{0S} \cdot \sqrt{130} = x_{0R} \cdot \sqrt{70}$$ --> Ortalamaları
    % da bulunan x0 olacak.

    % Ortalama x0 = 0.53e-3 idi. Bunu asimetrik dağıtıyoruz:
    % x0_S = 0.47e-3;  % Supply tarafı (0.47 mA)
    % x0_R = 0.64e-3;  % Return tarafı (0.64 mA)
    
    x0_S = 0.46e-3 ;  % Supply tarafı (0.46 mA) --> bunu editledim
    x0_R = 0.64e-3 ;  % Return tarafı (0.64 mA)

    % x0_S = 0.53e-3;  % Supply tarafı (0.47 mA)
    % x0_R = 0.53e-3;  % Return tarafı (0.64 mA)

    K_tare = 2.345e-9; 
    
    % Güvenlik (Basınçlar)
    dPs1 = max(0, Ps - P1); dP1r = max(0, P1 - Pr);
    dPs2 = max(0, Ps - P2); dP2r = max(0, P2 - Pr);
    dPsr = max(0, Ps - Pr);

    if u >= 0
        % P_S -> P_1 (Supply Side - Ana Akış) -> x0_S kullan
        Q1_S = K * sqrt(dPs1) * (x0_S + u); 
        
        % P_1 -> P_R (Return Side - Sızıntı) -> x0_R kullan
        Q1_R = K * sqrt(dP1r) * (x0_R^2 / (x0_R + k*u)); 

        % P_S -> P_2 (Supply Side - Sızıntı) -> x0_S kullan
        Q2_S = K * sqrt(dPs2) * (x0_S^2 / (x0_S + k*u)); 
        
        % P_2 -> P_R (Return Side - Ana Akış) -> x0_R kullan
        Q2_R = K * sqrt(dP2r) * (x0_R + u);
    else
        % x < 0 durumu
        % Simetriyi korumak için x negatifken de Supply/Return rollerine göre
        % doğru x0'ı seçmeliyiz.
        
        % P_S -> P_1 (Supply Side - Sızıntı)
        Q1_S = K * sqrt(dPs1) * (x0_S^2 / (x0_S - k*u)); 
        
        % P_1 -> P_R (Return Side - Ana Akış)
        Q1_R = K * sqrt(dP1r) * (x0_R - u); 

        % P_S -> P_2 (Supply Side - Ana Akış)
        Q2_S = K * sqrt(dPs2) * (x0_S - u); 
        
        % P_2 -> P_R (Return Side - Sızıntı)
        Q2_R = K * sqrt(dP2r) * (x0_R^2 / (x0_R - k*u)); 
    end

    Q1 = Q1_S - Q1_R;
    Q2 = Q2_S - Q2_R;
    QR = Q1_R + (Q2_R) + K_tare * sqrt(dPsr); 
end

== matlab function phdMain/Nguyen Observer/Nguyen_Observer/phi_calc/MATLAB Function4 ==
  data: v input; F_stribeck output
function F_stribeck = fcn(v)


% close all 

% --- Geçiş Yumuşaklığı Parametresi ---
% Bu değer büyüdükçe 0'daki eğim azalır (daha eğimli geçer)
eps_smooth = 0.0223;
% eps_smooth = 0.015;

%%%
kv_p = 12; Fc_p = 25; Fs_p  = 383; tau_p = 0.016;
kv_n = 35; Fc_n = 7.5; Fs_n = 183; tau_n = 0.02016;
%%%


% Yumuşatılmış yön fonksiyonu (sign yerine tanh)
% Bu fonksiyon -1 ile 1 arasında yumuşak bir geçiş sağlar
smooth_sign = tanh(v ./ eps_smooth);

% Asimetrik katsayı vektörleri oluşturma
% Hızın yönüne göre katsayıları seçiyoruz
kv = (v >= 0)*kv_p + (v < 0)*kv_n;
Fc = (v >= 0)*Fc_p + (v < 0)*Fc_n;
Fs = (v >= 0)*Fs_p + (v < 0)*Fs_n;
tau = (v >= 0)*tau_p + (v < 0)*tau_n;
F_stribeck = (Fc .* smooth_sign) + (Fs .* smooth_sign .* exp(-abs(v./tau)));

== matlab function phdMain/EKF_Healthy/EKF_Discrete ==
  data: u_perc input; x_hat_out output; y_k input; Fd_est output; Qd_est output
function [x_hat_out, Fd_est, Qd_est] = sdre_6state_crio(u_perc, y_k)
%SDRE_6STATE_CRIO  Discrete 6-state Extended State Observer (ESO)
%  Fully Physical Formulation: A(x) contains internal dynamics.
%  f(x,u) contains physical flows and hard friction nonlinearities.
%  Includes x5 (Mismatched Mech Disturbance) and x6 (Matched Hyd Disturbance).
%
%  States:  x = [pos(m), vel(m/s), PA(Pa), PB(Pa), Fd(N), Qd(m^3/s)]
%  Inputs:  u_k   - valve spool displacement command [m] (max 25e-5)
%           y_k   - [pos_m; PA_Pa; PB_Pa]  (measurements)
%           Ps_k  - supply pressure [Pa]
%           Pr_k  - return pressure [Pa]
%  Outputs: x_hat_out - [pos; vel; PA; PB; Fd; Qd] state estimate
%           Fd_est    - Estimated mechanical load/friction mismatch [N]
%           Qd_est    - Estimated hydraulic internal leakage/valve mismatch [m^3/s]
%#codegen

%% ── PERSISTENT STATE ─────────────────────────────────────────────────────
persistent x_hat P_k initialized;

%% ── SYSTEM PARAMETERS ────────────────────────────────────────────────────
M       = 3.4;
d_p     = 34e-3;   
d_r     = 30e-3;
A_c     = pi/4*(d_p^2 - d_r^2);   
V_dead  = 1.5315e-5;
V_0     = A_c*(190.16e-3/2) + V_dead;   
C_t     = 3.9933e-13;
beta    = 1.6e9;
Ps_k    = 200e5; 
Pr_k    = 4e5; 

% Valve Parameters
K_sv    = 3.34e-6;
k_sv    = 1.82709080;
x0_S    = 0.46e-3;
x0_R    = 0.64e-3;
K_tare  = 2.345e-9; 
u_k     = u_perc * 25e-5; % Scale % to 25mA
% Observer design
dt          = 1e-3;
alpha_Fd    = 1e-2;   % Mechanical disturbance decay factor
alpha_Qd    = 0.2;    % Hydraulic disturbance decay factor

% Tuning Matrices (Optimized for robust model-measurement balance)
% Q_d6 = diag([1E-12,... %x1
%              1E-5,... %x2
%              1E0, 1E0, ... %x3 x4
%              1E-7, ... %Fd
%              1e-3]); %Qd

% Q_d6: x5 serbest bırakıldı, x2 esnetildi
% Q_d6: Kinematiği katılaştırıp, x5'i öğrenmeye açıyoruz
Q_d6 = diag([1E-14, ... % x1: dx1/dt = x2 ilişkisi KUSURSUZ kabul edilsin (Titremeyi bu önler)
             5E-5,  ... % x2: Hızın tepe noktalarına çıkış izni
             1E0,   ... % x3: PA
             1E0,   ... % x4: PB
             1E-2,  ... % x5: Fd_est ÇOK hızlı güncellensin (Asimetrik sürtünmeyi anında öğrensin)
             1E-3]);... % x6: Qd_est

% Tuning Matrices (Optimized for robust model-measurement balance)
% Q_d6 = diag([1E-12,... %x1
%              1E-6,... %x2
%              1E0, 1E0, ... %x3 x4
%              1E-3, ... %Fd
%              1e-3]); %Qd

R_m6 = diag([1E-10, 5E-2, 5E-2]);

% Scaling (Qd is ~1e-5 m^3/s, so we scale by 1e5 to keep it ~1.0)
SC6  = [1; 1; 1e-7; 1e-7; 1e-2; 1e5];
SCI6 = [1; 1; 1e7;  1e7;  1e2;  1e-5]; % <--- Son eleman 1e-5 OLMAK ZORUNDA
I6   = eye(6);
C_sc6 = [1 0 0 0 0 0; 
         0 0 1 0 0 0; 
         0 0 0 1 0 0];

%% ── INITIALIZATION ───────────────────────────────────────────────────────
if isempty(initialized)
    % Initialize 6 states
    x_hat = [y_k(1); 0; y_k(2); y_k(3); 0; 0];
    P_k   = diag([1e-6, 1e-4, 1e-6, 1e-6, 1e-4, 1e-6]);
    initialized = true;
end

%% ── STATE EXTRACTION ────────────────────────────────────────────────────
x1 = x_hat(1); % Position
x2 = x_hat(2); % Velocity
x3 = x_hat(3); % PA
x4 = x_hat(4); % PB

%% ── STEP 1: Asymmetric Friction (Linear/Nonlinear Split) ────────────────
% if x2 > 0
%     F_c = 6.93; F_s = 73.77; B_v = 33.96; v_st = 0.0372;
% else
%     F_c = 19.39; F_s = 52.45; B_v = 31.98; v_st = 0.0376;
% end
% 

% 
% % f6 vector component (Nonlinear Stribeck/Coulomb)
% if abs(x2) > 1e-6
%     F_nl = sign(x2) * ( F_c + (F_s - F_c)*exp(-(x2/v_st)^2) );
% else
%     F_nl = 0; 
% end

kv = 38;
% % A6 Matrix component (Linear Viscous Damping)
a22 = -kv / M;

F_nl = 0;



%% ── STEP 2: Robust Physical Valve Flows ─────────────────────────────────
% P_tol prevents zero derivative (inf gain) when pressure hits rails
P_tol = 0.1*1e5; % 0.1 bar tolerance


PA_c = max(Pr_k + P_tol, min(Ps_k - P_tol, x3));
PB_c = max(Pr_k + P_tol, min(Ps_k - P_tol, x4));

if u_k >= 0
    Q1_s = K_sv * sqrt(Ps_k - PA_c) * (x0_S + u_k);
    Q1_r = K_sv * sqrt(PA_c - Pr_k) * (x0_R^2 / (x0_R + k_sv*u_k));
    
    Q2_s = K_sv * sqrt(Ps_k - PB_c) * (x0_S^2 / (x0_S + k_sv*u_k)); 
    Q2_r = K_sv * sqrt(PB_c - Pr_k) * (x0_R + u_k);
else
    Q1_s = K_sv * sqrt(Ps_k - PA_c) * (x0_S^2 / (x0_S - k_sv*u_k));
    Q1_r = K_sv * sqrt(PA_c - Pr_k) * (x0_R - u_k);
    
    Q2_s = K_sv * sqrt(Ps_k - PB_c) * (x0_S - u_k);
    Q2_r = K_sv * sqrt(PB_c - Pr_k) * (x0_R^2 / (x0_R - k_sv*u_k));
end

Q1 = Q1_s - Q1_r; % Net flow into A
Q2 = Q2_s - Q2_r; % Net flow into B
% Q_return = Q1_R + Q2_R + K_tare * sqrt(Ps_k - Pr_k); 
%% ── STEP 3: State-Dependent Volumes (gamma) ─────────────────────────────
% Calculate instantaneous fluid stiffness
V_A = V_0 + A_c * x1;
V_B = V_0 - A_c * x1;

% Prevent volumes from dropping below zero geometrically
V_A = max(1e-6, V_A);
V_B = max(1e-6, V_B);

gamma_A = beta / V_A;
gamma_B = beta / V_B;

%% ── STEP 4: Build SDC Matrices (A6 and f6) ──────────────────────────────
% A6: Internal couplings and linear leakages + Disturbance Dynamics
A6 = [0,  1,               0,                 0,                0,          0;
      0,  a22,             A_c/M,            -A_c/M,            1/M,        0;
      0, -gamma_A*A_c,    -gamma_A*C_t,       gamma_A*C_t,      0,          gamma_A;
      0,  gamma_B*A_c,     gamma_B*C_t,      -gamma_B*C_t,      0,         -gamma_B;
      0,  0,               0,                 0,               -alpha_Fd,   0;
      0,  0,               0,                 0,                0,         -alpha_Qd];

% f6: External physical forces, flow inputs, and hard nonlinearities
f6 = [0;
      0;
      gamma_A * Q1;
      gamma_B * Q2; 
      0;
      0];

% Forward Euler Discrete Integration
A_d6 = I6 + dt * A6;   

%% ── STEP 5: Scale Transform ──────────────────────────────────────────────
A_d6_sc = (SC6 * SCI6') .* A_d6;   
x_sc    = SC6 .* x_hat;
f_sc    = SC6 .* f6;

%% ── STEP 6: Kalman Predict ───────────────────────────────────────────────
x_pred_sc = A_d6_sc * x_sc + dt * f_sc; 

P_pred = A_d6_sc * P_k * A_d6_sc' + Q_d6;
P_pred = 0.5*(P_pred + P_pred'); 

%% ── STEP 7: Innovation & Kalman Gain ─────────────────────────────────────
z_sc   = [SC6(1)*y_k(1); SC6(3)*y_k(2); SC6(4)*y_k(3)];
innov  = z_sc - C_sc6 * x_pred_sc;
S6     = C_sc6 * P_pred * C_sc6' + R_m6;
S6     = 0.5 * (S6 + S6');

if rcond(S6) < 1e-14
    S6 = S6 + 1e-12 * eye(3);
end

K6    = (P_pred * C_sc6') / S6;
IKH6  = I6 - K6 * C_sc6;
P_k   = IKH6 * P_pred * IKH6' + K6 * R_m6 * K6';
P_k   = 0.5 * (P_k + P_k');

%% ── STEP 8: Update & Output ──────────────────────────────────────────────
x_hat = SCI6 .* (x_pred_sc + K6 * innov);

% Hard physical clamp on updated pressures
x_hat(3) = max(0, min(Ps_k, x_hat(3)));
x_hat(4) = max(0, min(Ps_k, x_hat(4)));

% Map to outputs
x_hat_out = x_hat;
Fd_est    = x_hat(5);
Qd_est    = x_hat(6);

end

== matlab function phdMain/old/MATLAB Function2 ==
  data: xv input; Q1 output; P_P input; P_T input; P_A input; P_B input; Q2 output; Q_RETURN output
function [Q1, Q2, Q_RETURN] = fcn_Valve_Tamburrano_Hybrid( ...
    xv, P_P, P_T, P_A, P_B)

% SI units:
% xv [m], P_* [Pa], w,c,r [m], rho [kg/m^3], mu [Pa*s], Cd [-]
%
% Outputs:
%   Q_A, Q_B         : Port net flows [m^3/s]
%   Q_Leak_Total     : leakage indicator [m^3/s]
%   Q_return_lpm     : total return flow to return line [LPM]

%% 0) Checks

%%
k = 0.2; 
K = 1.7817e-6; 
x0 = 0.00099959586;

x = xv;
P_S = P_P;
P_A = P_A; 
P_B = P_B;
P_R = P_T;

K1_S = K;
K1_R = K; 
K2_S = K; 
K2_R = K; 

k1_s = k; 
k1_r = k; 
k2_s = k; 
k2_r = k; 

%% 
if x >= 0
        % For control port 1
        Q1_S = K1_S * sqrt(abs(P_S - P_A)) * (x0 + x) * sign(P_S - P_A);
        Q1_R = K1_R * sqrt(abs(P_A - P_R)) * (x0^2) * ((x0 + k1_r*x)^-1) *sign(P_A - P_R);

        % For control port 2
        Q2_S = K2_S * sqrt(abs(P_S - P_B)) * (x0^2) * ((x0 + k2_s*x)^-1) *sign((P_S - P_B)); 
        Q2_R = K2_R * sqrt(abs(P_B - P_R)) * (x0 + x) * sign((P_B - P_R)); 
else 
        % For control port 1
        Q1_S = K1_S * sqrt(abs(P_S - P_A)) * (x0^2) * ((x0 - k1_s*x)^-1) * sign(P_S - P_A);
        Q1_R = K1_R * sqrt(abs(P_A - P_R)) * (x0 - x) * sign(P_A - P_R);

        % For control port 2
        Q2_S = K2_S * sqrt(abs(P_S - P_B)) * (x0 - x) * sign(P_S - P_B); 
        Q2_R = K2_R * sqrt(abs(P_B - P_R)) * (x0^2) * ((x0 - k2_r*x)^-1)* sign(P_B - P_R); 
end 

Q1 = Q1_S - Q1_R; 
Q2 = Q2_S - Q2_R; 

Q_RETURN = Q1_R + Q2_R;

== matlab function phdMain/Plant/Subsystem1/MATLAB Function ==
  data: Q1 output; Q2 output; x input; Ps input; Pr input; P1 input; P2 input; K input; k input; QR output
function [Q1, Q2, QR] = fcn(x, Ps, Pr, P1, P2, K, k)
    % x0 parametresini girişten kaldırdık, içeride asimetrik tanımlayacağız.
    
    % --- ASİMETRİK SIZINTI AYARLARI ---
    % Hedef: P_null = 70 bar (Ps=210 bar iken)
    % Bu dengeyi sağlamak için Return tarafı açıklığı daha büyük olmalı.

    % --- GÜNCELLENMİŞ ASİMETRİK SIZINTI AYARLARI ---
    % Hedef: Ps=200 bar, Pr=4.5 bar iken yaklaşık 70-75 bar denge basıncı
    % $$x_{0S} \cdot \sqrt{130} = x_{0R} \cdot \sqrt{70}$$ --> Ortalamaları
    % da bulunan x0 olacak.

    % Ortalama x0 = 0.53e-3 idi. Bunu asimetrik dağıtıyoruz:
    % x0_S = 0.47e-3;  % Supply tarafı (0.47 mA)
    % x0_R = 0.64e-3;  % Return tarafı (0.64 mA)
    
    x0_S = 0.46e-3 ;  % Supply tarafı (0.46 mA) --> bunu editledim
    x0_R = 0.64e-3 ;  % Return tarafı (0.64 mA)

    % x0_S = 0.53e-3;  % Supply tarafı (0.47 mA)
    % x0_R = 0.53e-3;  % Return tarafı (0.64 mA)

    K_tare = 2.345e-9; 
    
    % Güvenlik (Basınçlar)
    dPs1 = max(0, Ps - P1); dP1r = max(0, P1 - Pr);
    dPs2 = max(0, Ps - P2); dP2r = max(0, P2 - Pr);
    dPsr = max(0, Ps - Pr);

    if x >= 0
        % P_S -> P_1 (Supply Side - Ana Akış) -> x0_S kullan
        Q1_S = K * sqrt(dPs1) * (x0_S + x); 
        
        % P_1 -> P_R (Return Side - Sızıntı) -> x0_R kullan
        Q1_R = K * sqrt(dP1r) * (x0_R^2 / (x0_R + k*x)); 

        % P_S -> P_2 (Supply Side - Sızıntı) -> x0_S kullan
        Q2_S = K * sqrt(dPs2) * (x0_S^2 / (x0_S + k*x)); 
        
        % P_2 -> P_R (Return Side - Ana Akış) -> x0_R kullan
        Q2_R = K * sqrt(dP2r) * (x0_R + x);
    else
        % x < 0 durumu
        % Simetriyi korumak için x negatifken de Supply/Return rollerine göre
        % doğru x0'ı seçmeliyiz.
        
        % P_S -> P_1 (Supply Side - Sızıntı)
        Q1_S = K * sqrt(dPs1) * (x0_S^2 / (x0_S - k*x)); 
        
        % P_1 -> P_R (Return Side - Ana Akış)
        Q1_R = K * sqrt(dP1r) * (x0_R - x); 

        % P_S -> P_2 (Supply Side - Ana Akış)
        Q2_S = K * sqrt(dPs2) * (x0_S - x); 
        
        % P_2 -> P_R (Return Side - Sızıntı)
        Q2_R = K * sqrt(dP2r) * (x0_R^2 / (x0_R - k*x)); 
    end

    Q1 = Q1_S - Q1_R;
    Q2 = Q2_S - Q2_R;
    QR = Q1_R + (Q2_R) + K_tare * sqrt(dPsr); 
end

== matlab function phdMain/Plant/Cylinder_Dynamics/Subsystem1/MATLAB Function1 ==
  data: x input; F_end output; x_dot input; xmin input; xmax input; k_end input; v_lock input
function F_end = endstop_force_simple(x, x_dot, xmin, xmax, k_end, v_lock)
%#codegen
% Very stable end-stop with velocity locking
% Minimal oscillation, solver-friendly

% v_lock : velocity below which motion is considered zero (m/s)
% Typical: 1e-3 … 5e-3

F_end = 0.0;
ccc = 1e6; 
% ---- LOWER STOP ----
if x <= xmin
    % spring force
    F_end = k_end * (xmin - x);

    % velocity lock (kill oscillation)
    if x_dot < v_lock
        F_end = F_end - ccc * x_dot;   % artificial strong damping
    end
end

% ---- UPPER STOP ----
if x >= xmax
    % spring force
    F_end = -k_end * (x - xmax);

    % velocity lock
    if x_dot > -v_lock
        F_end = F_end - ccc * x_dot;
    end
end

== matlab function phdMain/old/Flow_Calc_WithLeak/MATLAB Function2 ==
  data: xv input; Q_A output; P_P input; P_T input; P_R input; P_A input; P_B input; w input; Q_B output; Q_Leak_Total_lpm output; c input; r input; rho input; mu input; Cd input; bias_P_dynamic input; bias_T_dynamic input; Q_return_model_lpm output; x_leak input
function [Q_A, Q_B, Q_Leak_Total_lpm, Q_return_model_lpm] = fcn_Valve_Tamburrano_Hybrid( ...
    xv, P_P, P_T, P_R, P_A, P_B, w, c, r, rho, mu, Cd, ...
    bias_P_dynamic, bias_T_dynamic, x_leak)

% SI units:
% xv [m], P_* [Pa], w,c,r [m], rho [kg/m^3], mu [Pa*s], Cd [-]
%
% Outputs:
%   Q_A, Q_B         : Port net flows [m^3/s]
%   Q_Leak_Total     : leakage indicator [m^3/s]
%   Q_return_lpm     : total return flow to return line [LPM]

%% 0) Checks
if c <= 0 || w <= 0 || rho <= 0 || mu <= 0 || Cd <= 0 || r < 0
    error('SI parametreler: w>0, c>0, r>=0, rho>0, mu>0, Cd>0 olmalı.');
end

%% 1) Tamburrano Eq.(19) -> l_eff (r,c'den)
if r == 0
    l_eff = c;
else
    y = (-(2*c + 4*r) + sqrt((2*c + 4*r)^2 + 16*r^2)) / 2; % y=l-c
    y = max(y, 0);
    l_eff = c + y;
end

%% 2) Tamburrano Eq.(18): laminer leakage conductance
K_lam_base = (pi * w * (l_eff^2)) / (32 * mu);  % [m^3/(s*Pa)]

%% 3) Static/Dynamic bias (pressure-holding + dynamic offset reduction)
transition_width = 20.5e-5;           % [m] (tune)
move_factor = tanh(abs(xv)/transition_width);

% --- Static
bias_P_static = 0.460;
bias_T_static = 0.9050;

% --- Interpolate to dynamic values ---
leak_bias_P = bias_P_static*(1-move_factor) + bias_P_dynamic*move_factor;
leak_bias_T = bias_T_static*(1-move_factor) + bias_T_dynamic*move_factor;


leak_bias_P = max(leak_bias_P, 0);
leak_bias_T = max(leak_bias_T, 0);



%% 4) Null-weighting for laminar leakage (keeps M-profile in motion)
% x_leak = 2.0e-4;                      % [m] (tune)
g = exp(-(abs(xv)/x_leak)^2);

%% 5) Metering areas
A_open = w * abs(xv);

if xv >= 0
    Area_PA = A_open;  Area_AT = 0;
    Area_PB = 0;       Area_BT = A_open;
else
    Area_PA = 0;       Area_AT = A_open;
    Area_PB = A_open;  Area_BT = 0;
end

%% 6) ΔP
dP_PA = (P_P - P_A);
dP_AT = (P_A - P_T);
dP_PB = (P_P - P_B);
dP_BT = (P_B - P_T);

%% 7) Orifice flows (Eq.7–10)
Q_PA_or = Cd * Area_PA * sign(dP_PA) * sqrt(2/rho * abs(dP_PA));
Q_AT_or = Cd * Area_AT * sign(dP_AT) * sqrt(2/rho * abs(dP_AT));
Q_PB_or = Cd * Area_PB * sign(dP_PB) * sqrt(2/rho * abs(dP_PB));
Q_BT_or = Cd * Area_BT * sign(dP_BT) * sqrt(2/rho * abs(dP_BT));

%% 8) Laminar leakage flows (Eq.18) with bias + null-weighting g
Q_PA_lam = (K_lam_base * leak_bias_P) * dP_PA;
Q_PB_lam = (K_lam_base * leak_bias_P) * dP_PB;
Q_AT_lam = (K_lam_base * leak_bias_T) * dP_AT;
Q_BT_lam = (K_lam_base * leak_bias_T) * dP_BT;

Q_PA = Q_PA_or + g * Q_PA_lam;
Q_PB = Q_PB_or + g * Q_PB_lam;
Q_AT = Q_AT_or + g * Q_AT_lam;
Q_BT = Q_BT_or + g * Q_BT_lam;

%% 9) Port net flows
Q_A = Q_PA - Q_AT;
Q_B = Q_PB - Q_BT;

%% 10) Return-line measured flow (valve-to-tank + extra bypass)
% Valve return to tank/return line:
Q_return_valve = max(Q_AT,0) + max(Q_BT,0);  % [m^3/s]

% C_bypass ≈ 6.43e-13 m^3/(s*Pa)
C_bypass = 6.43e-13; %1.628161 * 0.6*1.1;
Q_bypass = C_bypass * max(P_P - P_R, 0);     % [m^3/s]

Q_return_total = Q_return_valve + Q_bypass;
Q_return_model_lpm   = 60000 * Q_return_total;

%% 11) Leakage indicator (trend)
Q_Leak_Total = 0.5*(abs(Q_PA) + abs(Q_PB) + abs(Q_AT) + abs(Q_BT)) ...
              - 0.5*abs(Q_A + Q_B);
Q_Leak_Total_lpm = Q_Leak_Total * 60e3;
end
